simulink model "session2"  (R2018b)
settings: Solver=VariableStepAuto  StartTime=0.0  StopTime=10.0  RelTol=1e-3
libraries: simulink x2
settings Model: Creator=lenovo2  LastModifiedBy=lenovo2

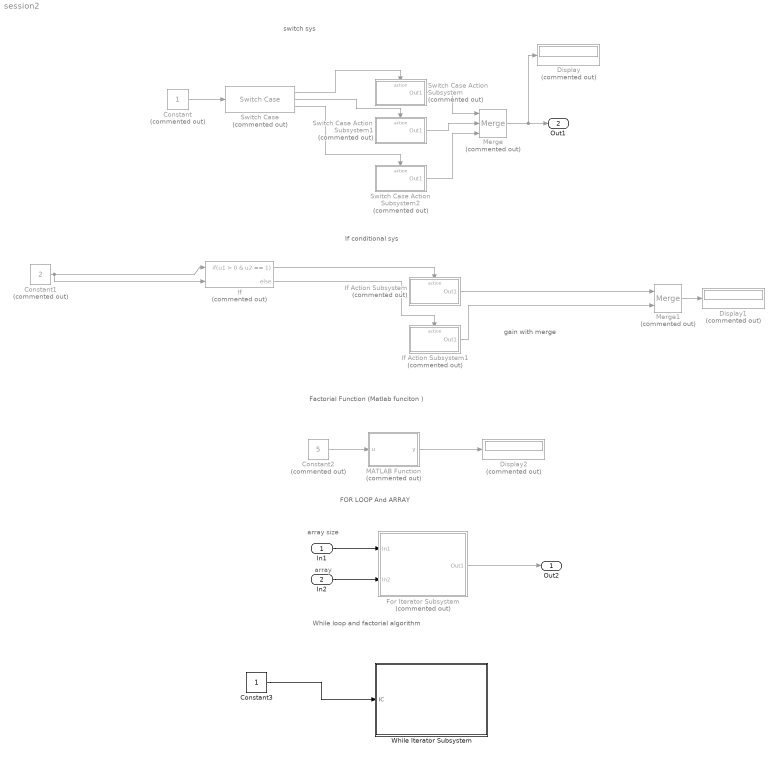
== system session2 ==
  note: While loop and factorial algorithm
  note: array
  note: array size
  note: FOR LOOP And ARRAY
  note: Factorial Function (Matlab funciton )
  note: gain with merge
  note: switch sys
  note: If conditional sys
  In1 : Inport  OutDataTypeStr=uint32
  In2 : Inport  Port=2  OutDataTypeStr=uint32  PortDimensions=5
  Constant : Constant  Commented=on
  Constant1 : Constant  Commented=on  Value=2
  Constant2 : Constant  Commented=on  Value=5
  Constant3 : Constant  OutDataTypeStr=int32
  Display : Display  Commented=on
  Display1 : Display  Commented=on
  Display2 : Display  Commented=on
  For Iterator Subsystem : Subsystem  Commented=on  TreatAsAtomicUnit=on
  If : If  Commented=on  NumInputs=2  IfExpression=u1 > 0 & u2 == 1
  If Action Subsystem : Subsystem  Commented=on  TreatAsAtomicUnit=on
  If Action Subsystem1 : Subsystem  Commented=on  TreatAsAtomicUnit=on
  MATLAB Function : MATLAB Function  Commented=on  TreatAsAtomicUnit=on
  Merge : Merge  Commented=on  Inputs=3
  Merge1 : Merge  Commented=on
  Switch Case : SwitchCase  Commented=on  CaseConditions={1,2}
  Switch Case Action Subsystem : Subsystem  Commented=on  TreatAsAtomicUnit=on
  Switch Case Action Subsystem1 : Subsystem  Commented=on  TreatAsAtomicUnit=on
  Switch Case Action Subsystem2 : Subsystem  Commented=on  TreatAsAtomicUnit=on
  While Iterator Subsystem : Subsystem  TreatAsAtomicUnit=on
  Out2 : Outport  OutDataTypeStr=uint32
  Out1 : Outport  Port=2
  wires:
  Switch Case/1 -> Switch Case Action Subsystem/Action
  Switch Case/2 -> Switch Case Action Subsystem1/Action
  Switch Case/3 -> Switch Case Action Subsystem2/Action
  Constant/1 -> Switch Case/1
  Switch Case Action Subsystem/1(Out1) -> Merge/1
  Switch Case Action Subsystem1/1(Out1) -> Merge/2
  Switch Case Action Subsystem2/1(Out1) -> Merge/3
  Merge/1 -> Display/1, Out1/1
  If/1 -> If Action Subsystem/Action
  If/2 -> If Action Subsystem1/Action
  If Action Subsystem/1(Out1) -> Merge1/1
  If Action Subsystem1/1(Out1) -> Merge1/2
  Merge1/1 -> Display1/1
  Constant1/1 -> If/2, If/1
  Constant2/1 -> MATLAB Function/1(u)
  MATLAB Function/1(y) -> Display2/1
  In1/1 -> For Iterator Subsystem/1(In1)
  In2/1 -> For Iterator Subsystem/2(In2)
  For Iterator Subsystem/1(Out1) -> Out2/1
  Constant3/1 -> While Iterator Subsystem/1(IC)

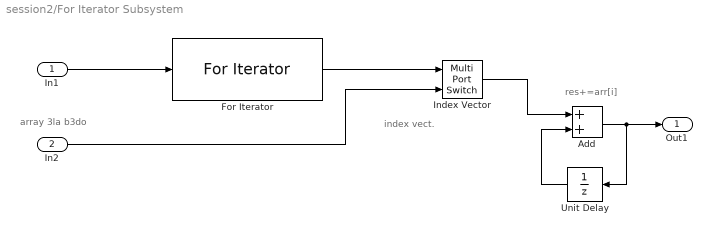
== system session2/For Iterator Subsystem ==
  note: res+=arr[i]
  note: index vect.
  note: array 3la b3do
  In1 : Inport
  In2 : Inport  Port=2
  Add : Sum
  For Iterator : ForIterator  IterationSource=external
  Index Vector : MultiPortSwitch  DataPortOrder=Zero-based contiguous  Inputs=1  zeroidx=on
  Unit Delay : UnitDelay  SampleTime=-1
  Out1 : Outport
  wires:
  In1/1 -> For Iterator/1
  In2/1 -> Index Vector/2
  Add/1 -> Out1/1, Unit Delay/1
  Index Vector/1 -> Add/1
  For Iterator/1 -> Index Vector/1
  Unit Delay/1 -> Add/2

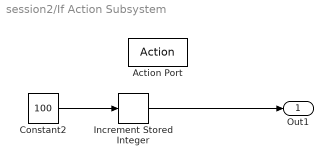
== system session2/If Action Subsystem ==
  Action Port : ActionPort  ActionType=then
  Constant2 : Constant  Value=100
  Increment Stored Integer : simulink/Additional Math & Discrete/Additional Math: Increment - Decrement/Increment Stored Integer
      settings: SourceProductName=Simulink
  Out1 : Outport
  wires:
  Constant2/1 -> Increment Stored Integer/1
  Increment Stored Integer/1 -> Out1/1

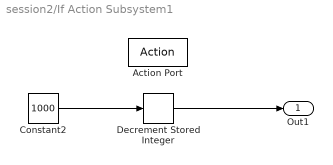
== system session2/If Action Subsystem1 ==
  Action Port : ActionPort  ActionType=else
  Constant2 : Constant  Value=1000
  Decrement Stored Integer : simulink/Additional Math & Discrete/Additional Math: Increment - Decrement/Decrement Stored Integer
      settings: SourceProductName=Simulink  SourceProductBaseCode=SL
  Out1 : Outport
  wires:
  Constant2/1 -> Decrement Stored Integer/1
  Decrement Stored Integer/1 -> Out1/1

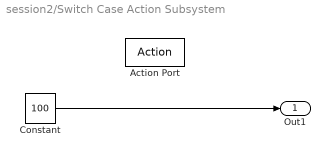
== system session2/Switch Case Action Subsystem ==
  Action Port : ActionPort  ActionType=case
  Constant : Constant  Value=100
  Out1 : Outport
  wires:
  Constant/1 -> Out1/1

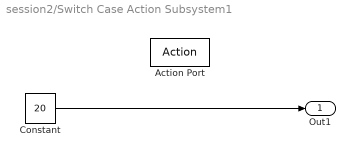
== system session2/Switch Case Action Subsystem1 ==
  Action Port : ActionPort  ActionType=case
  Constant : Constant  Value=20
  Out1 : Outport
  wires:
  Constant/1 -> Out1/1

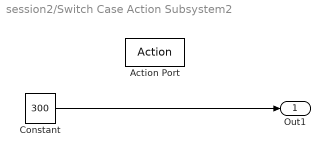
== system session2/Switch Case Action Subsystem2 ==
  Action Port : ActionPort  ActionType=default
  Constant : Constant  Value=300
  Out1 : Outport
  wires:
  Constant/1 -> Out1/1

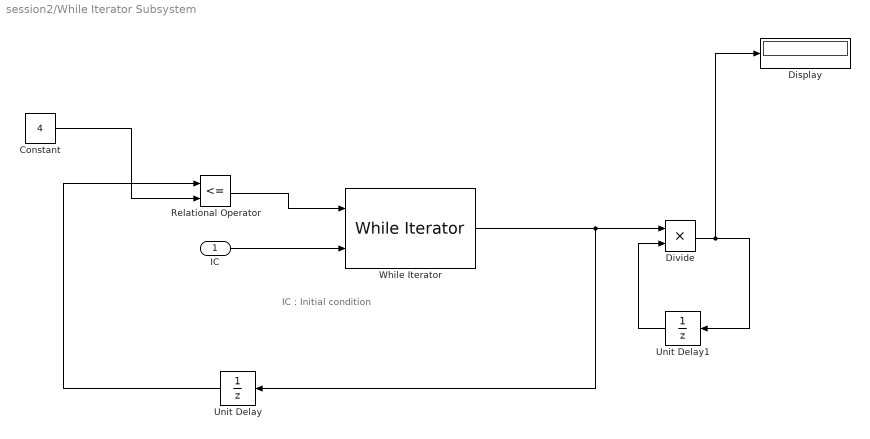
== system session2/While Iterator Subsystem ==
  note: IC : Initial condition
  IC : Inport  OutDataTypeStr=int32
  Constant : Constant  Value=4  OutDataTypeStr=int32
  Display : Display
  Divide : Product  Inputs=**  OutDataTypeStr=int32
  Relational Operator : RelationalOperator  Operator=<=  OutDataTypeStr=boolean  RndMeth=Simplest
  Unit Delay : UnitDelay  InitialCondition=1  SampleTime=-1
  Unit Delay1 : UnitDelay  InitialCondition=1  SampleTime=-1
  While Iterator : WhileIterator  MaxIters=4  ResetStates=reset  ShowIterationPort=on
  wires:
  IC/1 -> While Iterator/2
  Relational Operator/1 -> While Iterator/1
  While Iterator/1 -> Divide/1, Unit Delay/1
  Divide/1 -> Unit Delay1/1, Display/1
  Unit Delay/1 -> Relational Operator/1
  Constant/1 -> Relational Operator/2
  Unit Delay1/1 -> Divide/2

== matlab function session2/MATLAB Function ==
  data: u input; y output
function y = fcn(u)
fact = 1;
for i = 1 : u
    fact = i * fact ;
end
    
y = fact ;
